simulink subsystem "model_inductance_L2"  (R2024a)
settings: Solver=VariableStepAuto  StartTime=0.0  StopTime=10.0  RelTol=1e-3
values from neighbouring files (symbols this model uses):
  d = 0.20    (= 0.2)    [maglev_parameters.m]
  r = 0.020    (= 0.02)    [maglev_parameters.m]
settings Model: Creator=Bocchio  LastModifiedBy=Bocchio

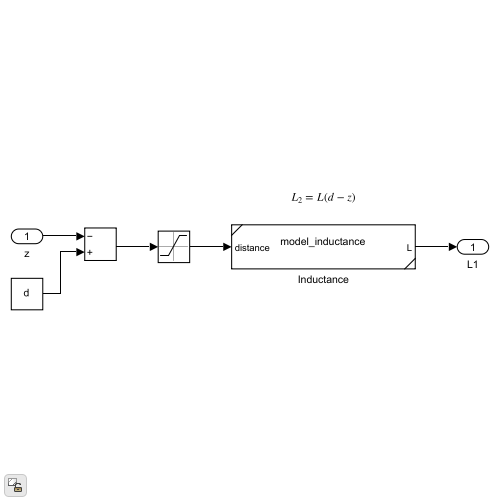
[thumbnail: Simulink's stored preview of the top-level diagram]
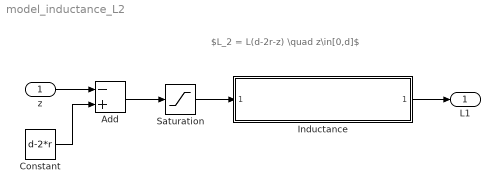
== system model_inductance_L2 ==
  note: $L_2 = L(d-2r-z) \quad z\in[0,d]$
  z : Inport
  Add : Sum  Inputs=-+
  Constant : Constant  Value=d-2*r
  Inductance : Subsystem  ReferencedSubsystem=model_inductance
  Saturation : Saturate  UpperLimit=d  LowerLimit=0
  L1 : Outport
  wires:
  Inductance/1 -> L1/1
  z/1 -> Add/1
  Constant/1 -> Add/2
  Add/1 -> Saturation/1
  Saturation/1 -> Inductance/1
